simulink model "Program_Counter_Increment"  (R2021a)
settings: Solver=VariableStepAuto  StartTime=0.0  StopTime=inf  RelTol=1e-3
libraries: dspsigops x1
settings Model: Creator=kbhar  LastModifiedBy=kbhar

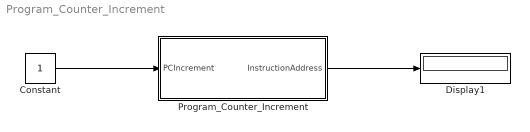
== system Program_Counter_Increment ==
  Constant : Constant
  Display1 : Display
  Program_Counter_Increment : Subsystem
  wires:
  Constant/1 -> Program_Counter_Increment/1(PCIncrement)
  Program_Counter_Increment/1(InstructionAddress) -> Display1/1

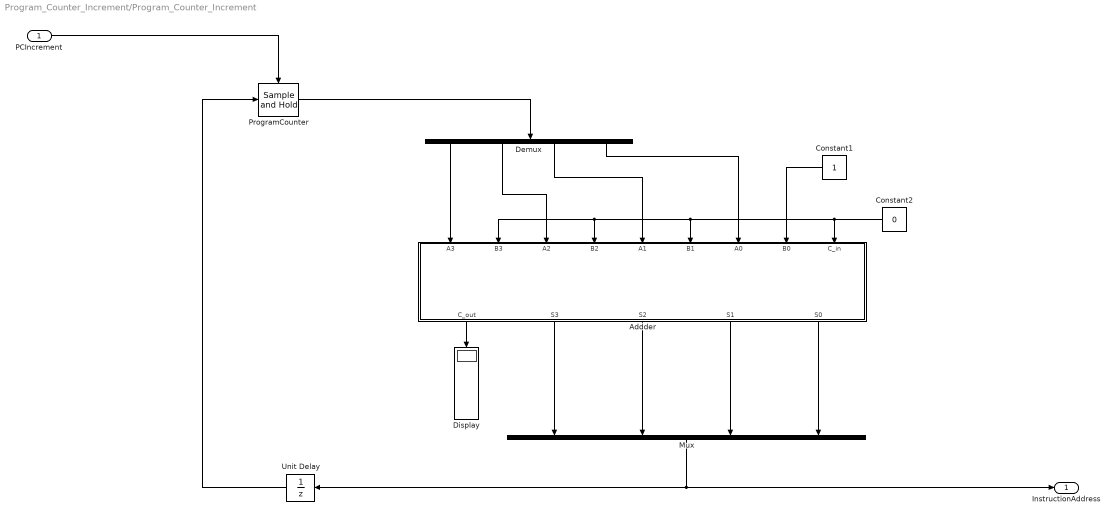
== system Program_Counter_Increment/Program_Counter_Increment ==
  PCIncrement : Inport
  Addder : Subsystem
  Constant1 : Constant
  Constant2 : Constant  Value=0
  Demux : Demux
  Display : Display
  Mux : Mux
  ProgramCounter : dspsigops/Sample and Hold  trig=Rising edge  initCond=[0 0 0 0]  latchinput=off
  Unit Delay : UnitDelay  SampleTime=-1  HasFrameUpgradeWarning=on
  InstructionAddress : Outport
  wires:
  Constant2/1 -> Addder/2(B3), Addder/4(B2), Addder/6(B1), Addder/9(C_in)
  Demux/3 -> Addder/5(A1)
  Mux/1 -> InstructionAddress/1, Unit Delay/1
  Addder/4(S1) -> Mux/3
  ProgramCounter/1 -> Demux/1
  Addder/1(C_out) -> Display/1
  Unit Delay/1 -> ProgramCounter/1
  Addder/5(S0) -> Mux/4
  Addder/3(S2) -> Mux/2
  Constant1/1 -> Addder/8(B0)
  Addder/2(S3) -> Mux/1
  Demux/2 -> Addder/3(A2)
  Demux/4 -> Addder/7(A0)
  Demux/1 -> Addder/1(A3)
  PCIncrement/1 -> ProgramCounter/Trigger

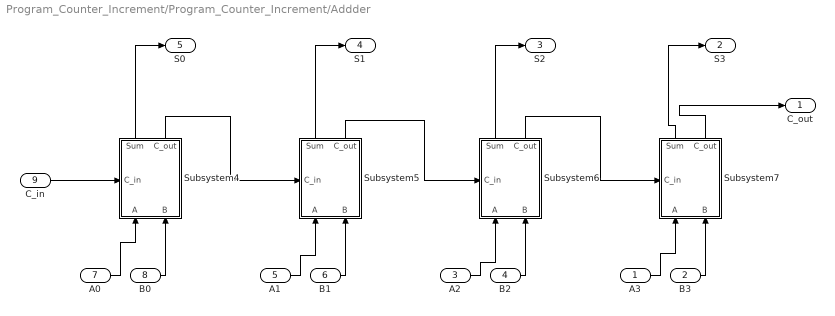
== system Program_Counter_Increment/Program_Counter_Increment/Addder ==
  A3 : Inport
  B3 : Inport  Port=2
  A2 : Inport  Port=3
  B2 : Inport  Port=4
  A1 : Inport  Port=5
  B1 : Inport  Port=6
  A0 : Inport  Port=7
  B0 : Inport  Port=8
  C_in : Inport  Port=9
  Subsystem4 : Subsystem
      settings: PortSchema="{\"entries\":[{\"content\":{\"sides\":[{\"content\":{\"connectorIds\":[\"In1\",\"In2\"]},\"type\":\"ConnectorPlacement.EquallySpacedRectSide\",\"uuid\":\"38d1d783-1e84-469f-b88f-34400794f458\"},{\"content\":{\"connectorIds\":[\"Out1\",\"Out2\"],\"side\":\"RIGHT\"},\"type\":\"ConnectorPlacement.EquallySpacedRectSide\",\"uuid\":\"9549b396-3b16-432f-9c12-dae7a5b8dc11\"},{\"content\":{\"connectorIds\":[\"In3\"],\"side\":\"TOP\"},\"type\":\"ConnectorPlacement.EquallySpacedRectSide\",\"uuid\":\"526a5790-86b3-4626-b4aa-b9520108ec40\"}]},\"type\":\"ConnectorPlacement.EquallySpacedConnector\",\"uuid\":\"b57ea0ad-738f-4734-9daa-a65058de1f48\"}],\"packageUris\":[\"http://schema.mathworks.com/mf0/Connector/R2020b\"],\"version\":\"1.0\"}"
  Subsystem5 : Subsystem
      settings: PortSchema="{\"entries\":[{\"content\":{\"sides\":[{\"content\":{\"connectorIds\":[\"In1\",\"In2\"]},\"type\":\"ConnectorPlacement.EquallySpacedRectSide\",\"uuid\":\"38d1d783-1e84-469f-b88f-34400794f458\"},{\"content\":{\"connectorIds\":[\"Out1\",\"Out2\"],\"side\":\"RIGHT\"},\"type\":\"ConnectorPlacement.EquallySpacedRectSide\",\"uuid\":\"9549b396-3b16-432f-9c12-dae7a5b8dc11\"},{\"content\":{\"connectorIds\":[\"In3\"],\"side\":\"TOP\"},\"type\":\"ConnectorPlacement.EquallySpacedRectSide\",\"uuid\":\"526a5790-86b3-4626-b4aa-b9520108ec40\"}]},\"type\":\"ConnectorPlacement.EquallySpacedConnector\",\"uuid\":\"b57ea0ad-738f-4734-9daa-a65058de1f48\"}],\"packageUris\":[\"http://schema.mathworks.com/mf0/Connector/R2020b\"],\"version\":\"1.0\"}"
  Subsystem6 : Subsystem
      settings: PortSchema="{\"entries\":[{\"content\":{\"sides\":[{\"content\":{\"connectorIds\":[\"In1\",\"In2\"]},\"type\":\"ConnectorPlacement.EquallySpacedRectSide\",\"uuid\":\"38d1d783-1e84-469f-b88f-34400794f458\"},{\"content\":{\"connectorIds\":[\"Out1\",\"Out2\"],\"side\":\"RIGHT\"},\"type\":\"ConnectorPlacement.EquallySpacedRectSide\",\"uuid\":\"9549b396-3b16-432f-9c12-dae7a5b8dc11\"},{\"content\":{\"connectorIds\":[\"In3\"],\"side\":\"TOP\"},\"type\":\"ConnectorPlacement.EquallySpacedRectSide\",\"uuid\":\"526a5790-86b3-4626-b4aa-b9520108ec40\"}]},\"type\":\"ConnectorPlacement.EquallySpacedConnector\",\"uuid\":\"b57ea0ad-738f-4734-9daa-a65058de1f48\"}],\"packageUris\":[\"http://schema.mathworks.com/mf0/Connector/R2020b\"],\"version\":\"1.0\"}"
  Subsystem7 : Subsystem
      settings: PortSchema="{\"entries\":[{\"content\":{\"sides\":[{\"content\":{\"connectorIds\":[\"In1\",\"In2\"]},\"type\":\"ConnectorPlacement.EquallySpacedRectSide\",\"uuid\":\"38d1d783-1e84-469f-b88f-34400794f458\"},{\"content\":{\"connectorIds\":[\"Out1\",\"Out2\"],\"side\":\"RIGHT\"},\"type\":\"ConnectorPlacement.EquallySpacedRectSide\",\"uuid\":\"9549b396-3b16-432f-9c12-dae7a5b8dc11\"},{\"content\":{\"connectorIds\":[\"In3\"],\"side\":\"TOP\"},\"type\":\"ConnectorPlacement.EquallySpacedRectSide\",\"uuid\":\"526a5790-86b3-4626-b4aa-b9520108ec40\"}]},\"type\":\"ConnectorPlacement.EquallySpacedConnector\",\"uuid\":\"b57ea0ad-738f-4734-9daa-a65058de1f48\"}],\"packageUris\":[\"http://schema.mathworks.com/mf0/Connector/R2020b\"],\"version\":\"1.0\"}"
  C_out : Outport
  S3 : Outport  Port=2
  S2 : Outport  Port=3
  S1 : Outport  Port=4
  S0 : Outport  Port=5
  wires:
  Subsystem5/2(C_out) -> Subsystem6/3(C_in)
  Subsystem5/1(Sum) -> S1/1
  Subsystem7/2(C_out) -> C_out/1
  B1/1 -> Subsystem5/2(B)
  Subsystem6/2(C_out) -> Subsystem7/3(C_in)
  A1/1 -> Subsystem5/1(A)
  A2/1 -> Subsystem6/1(A)
  Subsystem4/2(C_out) -> Subsystem5/3(C_in)
  B0/1 -> Subsystem4/2(B)
  B3/1 -> Subsystem7/2(B)
  B2/1 -> Subsystem6/2(B)
  A0/1 -> Subsystem4/1(A)
  A3/1 -> Subsystem7/1(A)
  Subsystem6/1(Sum) -> S2/1
  C_in/1 -> Subsystem4/3(C_in)
  Subsystem4/1(Sum) -> S0/1
  Subsystem7/1(Sum) -> S3/1

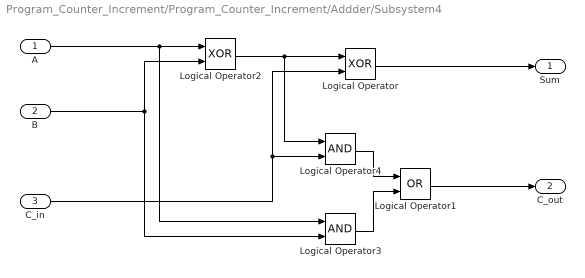
== system Program_Counter_Increment/Program_Counter_Increment/Addder/Subsystem4 ==
  A : Inport
  B : Inport  Port=2
  C_in : Inport  Port=3
  Logical Operator : Logic  Operator=XOR  AllPortsSameDT=off  OutDataTypeStr=boolean
  Logical Operator1 : Logic  Operator=OR  AllPortsSameDT=off  OutDataTypeStr=boolean
  Logical Operator2 : Logic  Operator=XOR  AllPortsSameDT=off  OutDataTypeStr=boolean
  Logical Operator3 : Logic  AllPortsSameDT=off  OutDataTypeStr=boolean
  Logical Operator4 : Logic  AllPortsSameDT=off  OutDataTypeStr=boolean
  Sum : Outport
  C_out : Outport  Port=2
  wires:
  B/1 -> Logical Operator3/2, Logical Operator2/2
  A/1 -> Logical Operator3/1, Logical Operator2/1
  Logical Operator4/1 -> Logical Operator1/1
  Logical Operator/1 -> Sum/1
  Logical Operator2/1 -> Logical Operator4/1, Logical Operator/1
  C_in/1 -> Logical Operator4/2, Logical Operator/2
  Logical Operator3/1 -> Logical Operator1/2
  Logical Operator1/1 -> C_out/1

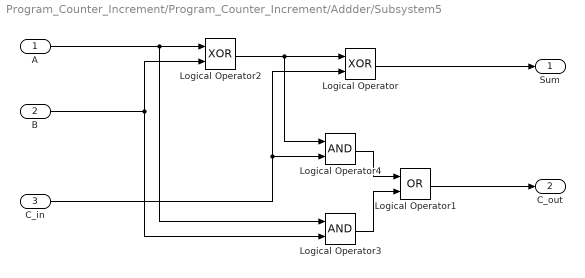
== system Program_Counter_Increment/Program_Counter_Increment/Addder/Subsystem5 ==
  A : Inport
  B : Inport  Port=2
  C_in : Inport  Port=3
  Logical Operator : Logic  Operator=XOR  AllPortsSameDT=off  OutDataTypeStr=boolean
  Logical Operator1 : Logic  Operator=OR  AllPortsSameDT=off  OutDataTypeStr=boolean
  Logical Operator2 : Logic  Operator=XOR  AllPortsSameDT=off  OutDataTypeStr=boolean
  Logical Operator3 : Logic  AllPortsSameDT=off  OutDataTypeStr=boolean
  Logical Operator4 : Logic  AllPortsSameDT=off  OutDataTypeStr=boolean
  Sum : Outport
  C_out : Outport  Port=2
  wires:
  B/1 -> Logical Operator3/2, Logical Operator2/2
  A/1 -> Logical Operator3/1, Logical Operator2/1
  Logical Operator4/1 -> Logical Operator1/1
  Logical Operator/1 -> Sum/1
  Logical Operator2/1 -> Logical Operator4/1, Logical Operator/1
  C_in/1 -> Logical Operator4/2, Logical Operator/2
  Logical Operator3/1 -> Logical Operator1/2
  Logical Operator1/1 -> C_out/1

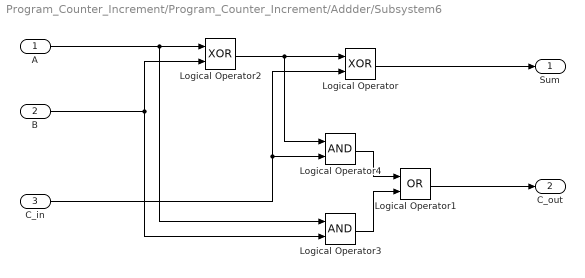
== system Program_Counter_Increment/Program_Counter_Increment/Addder/Subsystem6 ==
  A : Inport
  B : Inport  Port=2
  C_in : Inport  Port=3
  Logical Operator : Logic  Operator=XOR  AllPortsSameDT=off  OutDataTypeStr=boolean
  Logical Operator1 : Logic  Operator=OR  AllPortsSameDT=off  OutDataTypeStr=boolean
  Logical Operator2 : Logic  Operator=XOR  AllPortsSameDT=off  OutDataTypeStr=boolean
  Logical Operator3 : Logic  AllPortsSameDT=off  OutDataTypeStr=boolean
  Logical Operator4 : Logic  AllPortsSameDT=off  OutDataTypeStr=boolean
  Sum : Outport
  C_out : Outport  Port=2
  wires:
  B/1 -> Logical Operator3/2, Logical Operator2/2
  A/1 -> Logical Operator3/1, Logical Operator2/1
  Logical Operator4/1 -> Logical Operator1/1
  Logical Operator/1 -> Sum/1
  Logical Operator2/1 -> Logical Operator4/1, Logical Operator/1
  C_in/1 -> Logical Operator4/2, Logical Operator/2
  Logical Operator3/1 -> Logical Operator1/2
  Logical Operator1/1 -> C_out/1

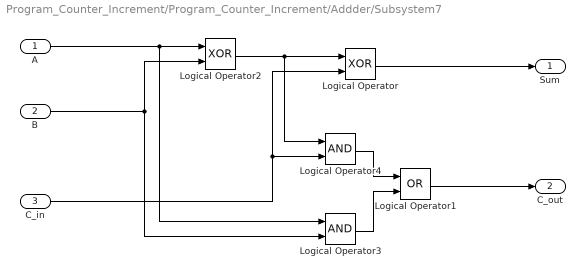
== system Program_Counter_Increment/Program_Counter_Increment/Addder/Subsystem7 ==
  A : Inport
  B : Inport  Port=2
  C_in : Inport  Port=3
  Logical Operator : Logic  Operator=XOR  AllPortsSameDT=off  OutDataTypeStr=boolean
  Logical Operator1 : Logic  Operator=OR  AllPortsSameDT=off  OutDataTypeStr=boolean
  Logical Operator2 : Logic  Operator=XOR  AllPortsSameDT=off  OutDataTypeStr=boolean
  Logical Operator3 : Logic  AllPortsSameDT=off  OutDataTypeStr=boolean
  Logical Operator4 : Logic  AllPortsSameDT=off  OutDataTypeStr=boolean
  Sum : Outport
  C_out : Outport  Port=2
  wires:
  B/1 -> Logical Operator3/2, Logical Operator2/2
  A/1 -> Logical Operator3/1, Logical Operator2/1
  Logical Operator4/1 -> Logical Operator1/1
  Logical Operator/1 -> Sum/1
  Logical Operator2/1 -> Logical Operator4/1, Logical Operator/1
  C_in/1 -> Logical Operator4/2, Logical Operator/2
  Logical Operator3/1 -> Logical Operator1/2
  Logical Operator1/1 -> C_out/1
